simulink model "chap02_02_47_mdl"  (R2013b)
settings: Solver=FixedStepDiscrete  StartTime=0.0  StopTime=10.0  FixedStep=0.5  RelTol=1e-3
settings Model: Creator=Administrator  LastModifiedBy=sunzx.fnst
settings SolverCC: AlgebraicLoopSolver=LineSearch

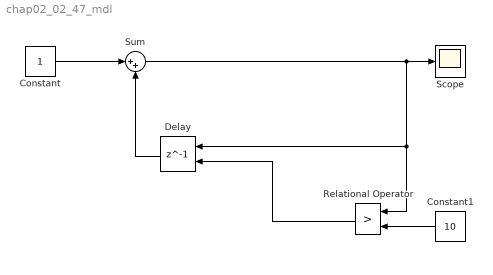
== system chap02_02_47_mdl ==
  Constant : Constant
  Constant1 : Constant  Value=10
  Delay : Delay  DelayLength=1  InitialCondition=0  ExternalReset=Level
      settings: InputPortMap=u0,r5
  Relational Operator : RelationalOperator  Operator=>  OutDataTypeStr=boolean  ZeroCross=off
  Scope : Scope
  Sum : Sum  Inputs=|++
  wires:
  Constant/1 -> Sum/1
  Sum/1 -> Relational Operator/1, Delay/1, Scope/1
  Delay/1 -> Sum/2
  Constant1/1 -> Relational Operator/2
  Relational Operator/1 -> Delay/2
